simulink model "demo_lqr_msd"  (R2025a)
settings: Solver=VariableStepAuto  StartTime=0.0  StopTime=3  RelTol=1e-3
settings Model: Creator=xing2  LastModifiedBy=xing2

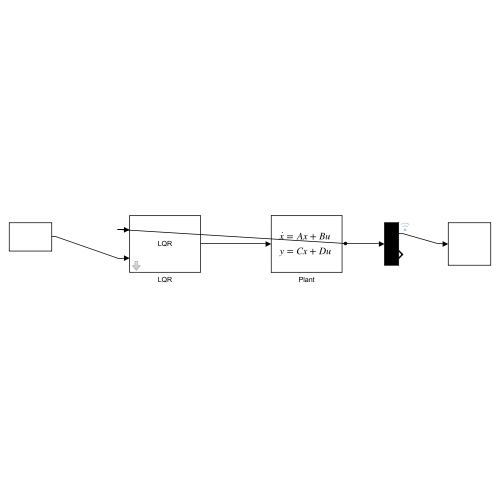
[thumbnail: Simulink's stored preview of the top-level diagram]
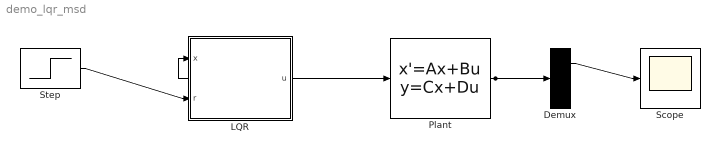
== system demo_lqr_msd ==
  Demux : Demux  Outputs=2
  LQR : Subsystem  mask{K_vec=[23.166247903554 7.02213372701576], Ki=0, UL=10, LL=-10}
      mask prompts: K_vec "K vector"; Ki "Ki (integral)"; UL "Upper Limit"; LL "Lower Limit"
      mask help: LQR State Feedback Controller with integral action
      mask Display: disp('LQR');
  Plant : StateSpace  A=[0 1;-10 -0.5]  B=[0;1]  C=eye(2)  D=[0;0]  InitialCondition=0
  Scope : Scope
  Step : Step  Time=0.5  SampleTime=0
  wires:
  Step/1 -> LQR/2(r)
  LQR/1(u) -> Plant/1
  Plant/1 -> Demux/1, LQR/1(x)
  Demux/1 -> Scope/1

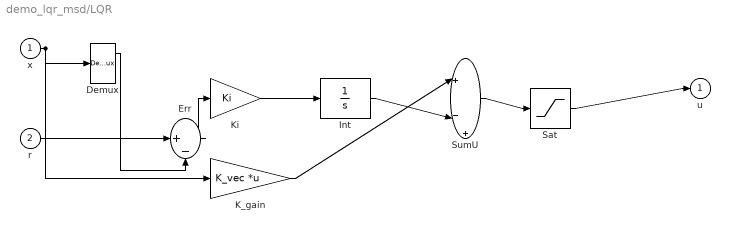
== system demo_lqr_msd/LQR ==
  x : Inport
  r : Inport  Port=2
  Demux : Demux  Outputs=2
  Err : Sum  Inputs=|+-
  Int : Integrator
  K_gain : Gain  Gain=K_vec  Multiplication=Matrix(K*u)
  Ki : Gain  Gain=Ki
  Sat : Saturate  UpperLimit=UL  LowerLimit=LL
  SumU : Sum  Inputs=|+-+
  u : Outport
  wires:
  Sat/1 -> u/1
  SumU/1 -> Sat/1
  Int/1 -> SumU/2
  K_gain/1 -> SumU/1
  Ki/1 -> Int/1
  Err/1 -> Ki/1
  Demux/1 -> Err/2
  r/1 -> Err/1
  x/1 -> K_gain/1, Demux/1
